simulink model "Gesamtmodell"  (R2017b)
settings: Solver=ode3  StartTime=0.0  StopTime=inf  FixedStep=dt  RelTol=1e-3  EnableMultiTasking=on
InitFcn:
  | Reglerauslegung
undefined symbols (not defined in the file or in its folder): aMax, aMaxPsi, Blindzeit, Com1, dt, K1, K2, K3, Kx, Ky, none, sigbuilder_block, Tx, Ty, vMax, vMaxPsi
libraries: xpcrtudplib x11, simulink x6, xpcutilitieslib x4, xpcseriallib x1, slrtlib x1
(part 1 of 4)
CloseFcn:
  | rtwprivate ssgencode ModelCloseRequest Robotino_Strecke_reall_2009
settings Model: SimulationMode=external  Creator=atlabor  LastModifiedBy=Robin
settings DataIOCC: SaveFormat=Array  SignalLoggingSaveFormat=ModelDataLogs
settings OptimizationCC: BlockReduction=off  OptimizeBlockIOStorage=off  BufferReuse=off  GlobalBufferReuse=off  ExpressionFolding=off  ExpressionDepthLimit=2147483647  LocalBlockOutputs=off  InitFltsAndDblsToZero=on  LifeSpan=inf
settings DebuggingCC: SaveWithParameterizedLinksMsg=none  UnderspecifiedInitializationDetection=Classic  MergeDetectMultiDrivingBlocksExec=none  SolverPrmCheckMsg=warning  FcnCallInpInsideContextMsg=warning  AllowSymbolicDim=off  StateNameClashWarn=warning  SFUnexpectedBacktrackingDiag=warning  SFNoUnconditionalDefaultTransitionDiag=warning  SFExecutionAtInitializationDiag=none
settings HardwareCC: ProdBitPerPointer=32  ProdBitPerSizeT=32  ProdBitPerPtrDiffT=32  ProdLargestAtomicFloat=None  ProdWordSize=32  ProdLongLongMode=on  ProdHWDeviceType=Generic->32-bit x86 compatible
settings ModelReferenceCC: PropagateSignalLabelsOutOfModel=off
settings SFSimCC: SimParseCustomCode=off
settings RTWCC: SystemTargetFile=slrt.tlc  TemplateMakefile=slrt_default_tmf  Description=Simulink Real-Time  CodeExecutionProfiling=on  RTWCompilerOptimization=on
settings CodeAppCC: StateflowObjectComments=on
settings ConfigComp: CovMetricSettings=dw  CovHtmlReporting=on  CovSaveCumulativeToWorkspaceVar=on  CovSaveSingleToWorkspaceVar=on  CovExternalEMLEnable=off  CovSFcnEnable=off

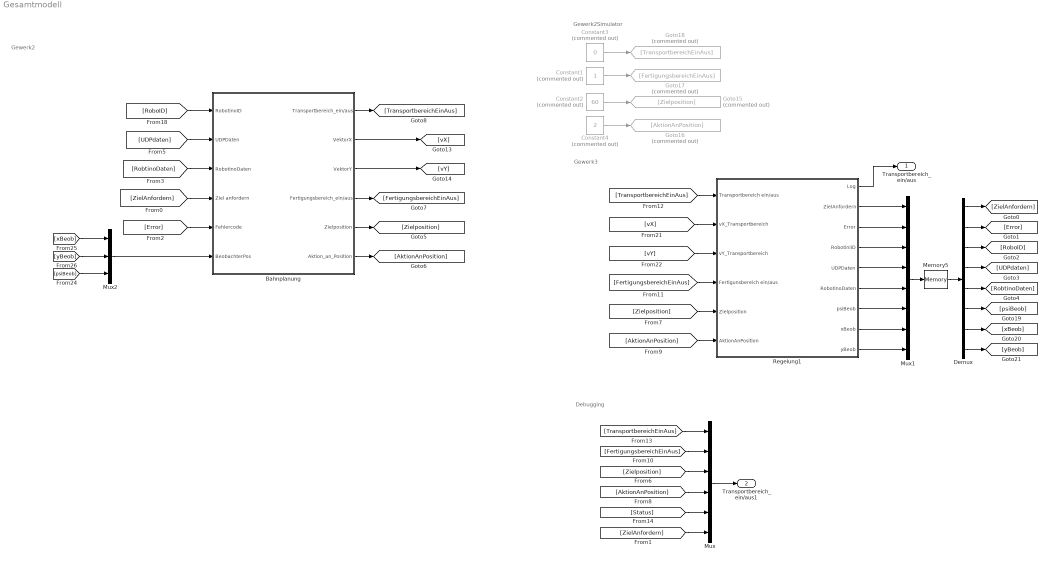
== system Gesamtmodell ==
  note: Gewerk2Simulator
  note: Gewerk3
  note: Gewerk2
  note: Debugging
  Bahnplanung : Subsystem
  Constant1 : Constant  Commented=on
  Constant2 : Constant  Commented=on  Value=60
  Constant3 : Constant  Commented=on  Value=0
  Constant4 : Constant  Commented=on  Value=2
  Demux : Demux  Outputs=8
  Goto15 : Goto  Commented=on  GotoTag=Zielposition
  Goto16 : Goto  Commented=on  GotoTag=AktionAnPosition
  Goto17 : Goto  Commented=on  GotoTag=FertigungsbereichEinAus
  Goto18 : Goto  Commented=on  GotoTag=TransportbereichEinAus
  Memory5 : Memory
  Mux : Mux  Inputs=6
  Mux1 : Mux  Inputs=8
  Mux2 : Mux  Inputs=3
  Regelung1 : Subsystem
  Transportbereich_ein/aus : Outport
  Transportbereich_ein/aus1 : Outport  Port=2
  wires:
  Regelung1/3(Error) -> Mux1/2
  Regelung1/6(RobotinoDaten) -> Mux1/5
  Regelung1/2(ZielAnfordern) -> Mux1/1
  Regelung1/4(RobotiniID) -> Mux1/3
  [ZielAnfordern] -> Mux/6
  Mux1/1 -> Memory5/1
  Demux/1 -> [ZielAnfordern]
  Demux/2 -> [Error]
  Memory5/1 -> Demux/1
  Demux/3 -> [RoboID]
  Demux/4 -> [UDPdaten]
  Regelung1/5(UDPDaten) -> Mux1/4
  Demux/5 -> [RobtinoDaten]
  [Zielposition] -> Mux/3
  [Zielposition] -> Regelung1/5(Zielposition)
  [AktionAnPosition] -> Mux/4
  [AktionAnPosition] -> Regelung1/6(AktionAnPosition)
  [FertigungsbereichEinAus] -> Mux/2
  [FertigungsbereichEinAus] -> Regelung1/4(Fertigunsbereich ein/aus)
  [TransportbereichEinAus] -> Regelung1/1(Transportbereich ein/aus)
  [TransportbereichEinAus] -> Mux/1
  [Status] -> Mux/5
  [vX] -> Regelung1/2(vX_Transportbereich)
  [vY] -> Regelung1/3(vY_Transportbereich)
  Constant3/1 -> Goto18/1
  Constant1/1 -> Goto17/1
  Constant2/1 -> Goto15/1
  Constant4/1 -> Goto16/1
  Regelung1/7(psiBeob) -> Mux1/6
  Regelung1/8(xBeob) -> Mux1/7
  Regelung1/9(yBeob) -> Mux1/8
  Demux/6 -> [psiBeob]
  Demux/7 -> [xBeob]
  Demux/8 -> [yBeob]
  [psiBeob] -> Mux2/3
  [xBeob] -> Mux2/1
  [yBeob] -> Mux2/2
  Regelung1/1(Log) -> Transportbereich_ein/aus/1
  Mux/1 -> Transportbereich_ein/aus1/1
  [UDPdaten] -> Bahnplanung/2(UDPDaten)
  [RobtinoDaten] -> Bahnplanung/3(RobotinoDaten)
  [ZielAnfordern] -> Bahnplanung/4(Ziel anfordern)
  [Error] -> Bahnplanung/5(Fehlercode)
  Mux2/1 -> Bahnplanung/6(BeobachterPos)
  Bahnplanung/1(Transportbereich_ein/aus) -> [TransportbereichEinAus]
  Bahnplanung/2(VektorX) -> [vX]
  Bahnplanung/3("VektorY ") -> [vY]
  Bahnplanung/4(Fertigungsbereich_ein/aus) -> [FertigungsbereichEinAus]
  Bahnplanung/5(Zielposition) -> [Zielposition]
  Bahnplanung/6(Aktion_an_Position) -> [AktionAnPosition]
  [RoboID] -> Bahnplanung/1(RobotinoID)

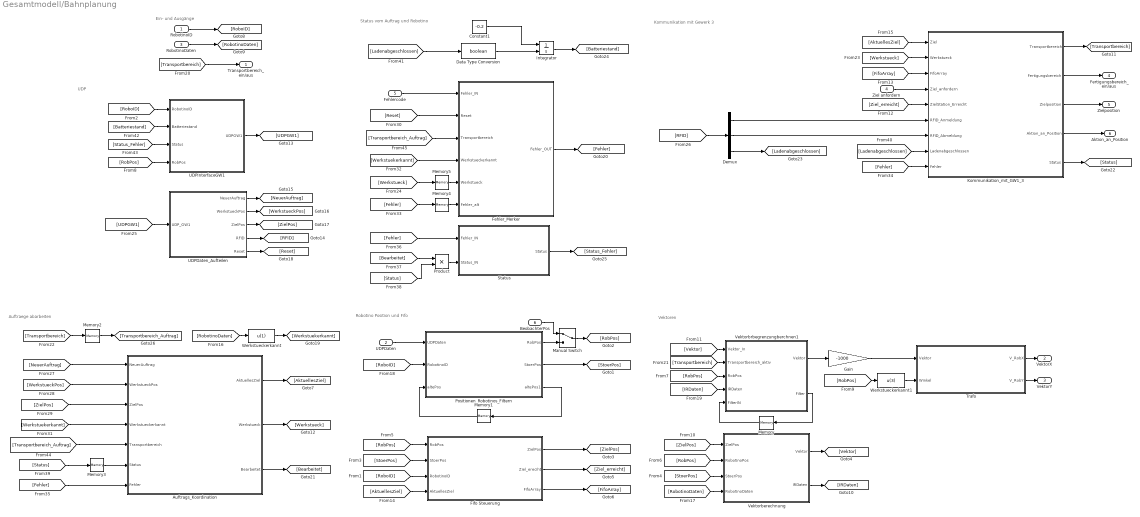
== system Gesamtmodell/Bahnplanung ==
  note: Ein- und Ausgänge
  note: Robotino Position und Fifo
  note: Status vom Auftrag und Robotino
  note: Auftraege abarbeiten
  note: Kommunikation mit Gewerk 3
  note: Vektoren
  note: UDP
  RobotinoID : Inport
  UDPDaten : Inport  Port=2  PortDimensions=56
  RobotinoDaten : Inport  Port=3
  Ziel anfordern : Inport  Port=4
  Fehlercode : Inport  Port=5
  BeobachterPos : Inport  Port=6
  Auftrags_Koordination : Stateflow chart  TreatAsAtomicUnit=on
  Constant1 : Constant  Value=-0.2
  Data Type Conversion : DataTypeConversion  OutDataTypeStr=boolean
  Demux : Demux  Outputs=3
  Fehler_Merker : MATLAB Function  TreatAsAtomicUnit=on
  Fifo Steuerung : Subsystem
  Gain : Gain  Gain=-1000
  Integrator : Integrator  ExternalReset=rising  InitialCondition=100  LimitOutput=on  UpperSaturationLimit=100  LowerSaturationLimit=0
  Kommunikation_mit_GW1_3 : Stateflow chart  TreatAsAtomicUnit=on
  Manual Switch : ManualSwitch
  Memory{,1..5} (6 alike) : Memory
  Positionen_Robotinos_Filtern : MATLAB Function  TreatAsAtomicUnit=on
  Product : Product
  Status : MATLAB Function  TreatAsAtomicUnit=on
  Trafo : MATLAB Function  Tag=Transformation_Global_auf_lokal  TreatAsAtomicUnit=on
  UDPDaten_Aufteilen : Subsystem
  UDPInterfaceGW1 : Subsystem
  Vektorberechnung : Subsystem
  Vektorbrbegrenzungberchnen1 : MATLAB Function  TreatAsAtomicUnit=on
  Werkstueckerkannt : Fcn  Expr=u(1)
  Werkstueckerkannt1 : Fcn  Expr=u(3)
  Transportbereich_ein/aus : Outport
  VektorX : Outport  Port=2  OutDataTypeStr=double
  "VektorY " : Outport  Port=3  OutDataTypeStr=double
  Fertigungsbereich_ein/aus : Outport  Port=4
  Zielposition : Outport  Port=5
  Aktion_an_Position : Outport  Port=6
  wires:
  Memory5/1 -> Fehler_Merker/5(Werkstueck)
  Memory4/1 -> Fehler_Merker/6(Fehler_alt)
  Data Type Conversion/1 -> Integrator/2
  Constant1/1 -> Integrator/1
  Fehlercode/1 -> Fehler_Merker/1(Fehler_IN)
  Memory1/1 -> Positionen_Robotinos_Filtern/3(altePos)
  Positionen_Robotinos_Filtern/3(altePos1) -> Memory1/1
  Memory/1 -> Vektorbrbegrenzungberchnen1/5(FilterIN)
  Demux/2 -> Kommunikation_mit_GW1_3/7(RFID_Abmeldung)
  Demux/1 -> Kommunikation_mit_GW1_3/6(RFID_Anmeldung)
  Ziel anfordern/1 -> Kommunikation_mit_GW1_3/4(Ziel_anfordern)
  Werkstueckerkannt1/1 -> Trafo/2(Winkel)
  BeobachterPos/1 -> Manual Switch/1
  Trafo/2(V_RobY) -> "VektorY "/1
  Trafo/1(V_RobX) -> VektorX/1
  Positionen_Robotinos_Filtern/1(RobPos) -> Manual Switch/2
  Gain/1 -> Trafo/1(Vektor)
  Vektorbrbegrenzungberchnen1/1(Vektor) -> Gain/1
  Kommunikation_mit_GW1_3/2(Fertigungsbereich) -> Fertigungsbereich_ein/aus/1
  Kommunikation_mit_GW1_3/4(Aktion_an_Position) -> Aktion_an_Position/1
  Kommunikation_mit_GW1_3/3(Zielposition) -> Zielposition/1
  UDPDaten/1 -> Positionen_Robotinos_Filtern/1(UDPDaten)
  [RoboID] -> Positionen_Robotinos_Filtern/2(RobotinoID)
  Memory3/1 -> Auftrags_Koordination/6(Status)
  RobotinoID/1 -> [RoboID]
  [RoboID] -> Fifo Steuerung/3(RobotinoID)
  [RoboID] -> UDPInterfaceGW1/1(RobotinoID)
  [StoerPos] -> Fifo Steuerung/2(StoerPos)
  [StoerPos] -> Vektorberechnung/3(StoerPos)
  Positionen_Robotinos_Filtern/2(StoerPos) -> [StoerPos]
  [RobPos] -> Fifo Steuerung/1(RobPos)
  [RobPos] -> Vektorberechnung/2(RobotinoPos)
  [RobPos] -> Vektorbrbegrenzungberchnen1/3(RobPos)
  [RobPos] -> UDPInterfaceGW1/4(RobPos)
  [RobPos] -> Werkstueckerkannt1/1
  Manual Switch/1 -> [RobPos]
  Fifo Steuerung/1(ZielPos) -> [ZielPos]
  [ZielPos] -> Vektorberechnung/1(ZielPos)
  Vektorberechnung/1(Vektor) -> [Vektor]
  [Vektor] -> Vektorbrbegrenzungberchnen1/1(Vektor_In)
  [Ziel_erreicht] -> Kommunikation_mit_GW1_3/5(ZielStation_Erreicht)
  Fifo Steuerung/2(Ziel_ereciht) -> [Ziel_erreicht]
  [FifoArray] -> Kommunikation_mit_GW1_3/3(FifoArray)
  Fifo Steuerung/3("FifoArray ") -> [FifoArray]
  [AktuellesZiel] -> Fifo Steuerung/4(AktuellesZiel)
  [AktuellesZiel] -> Kommunikation_mit_GW1_3/1(Ziel)
  Auftrags_Koordination/1(AktuellesZiel) -> [AktuellesZiel]
  [RobotinoDaten] -> Werkstueckerkannt/1
  [RobotinoDaten] -> Vektorberechnung/4(RobotinoDaten)
  RobotinoDaten/1 -> [RobotinoDaten]
  [IRDaten] -> Vektorbrbegrenzungberchnen1/4(IRDaten)
  Vektorberechnung/2(IRDaten) -> [IRDaten]
  [Transportbereich] -> Transportbereich_ein/aus/1
  [Transportbereich] -> Vektorbrbegrenzungberchnen1/2(Transportbereich_aktiv)
  [Transportbereich] -> Memory2/1
  Kommunikation_mit_GW1_3/1(Transportbereich) -> [Transportbereich]
  [Werkstueck] -> Kommunikation_mit_GW1_3/2(Werkstueck)
  [Werkstueck] -> Memory5/1
  Auftrags_Koordination/2(Werkstueck) -> [Werkstueck]
  [UDPGW1] -> UDPDaten_Aufteilen/1(UDP_GW1)
  UDPInterfaceGW1/1(UDPGW1) -> [UDPGW1]
  [RFID] -> Demux/1
  UDPDaten_Aufteilen/4(RFID) -> [RFID]
  [NeuerAuftrag] -> Auftrags_Koordination/1(NeuerAuftrag)
  UDPDaten_Aufteilen/1(NeuerAuftrag) -> [NeuerAuftrag]
  [WerkstueckPos] -> Auftrags_Koordination/2(WerkstueckPos)
  UDPDaten_Aufteilen/2(WerkstueckPos) -> [WerkstueckPos]
  [ZielPos] -> Auftrags_Koordination/3(ZielPos)
  UDPDaten_Aufteilen/3(ZielPos) -> [ZielPos]
  [Reset] -> Fehler_Merker/2(Reset)
  UDPDaten_Aufteilen/5(Reset) -> [Reset]
  [Werkstuekerkannt] -> Auftrags_Koordination/4(Werkstueckerkannt)
  [Werkstuekerkannt] -> Fehler_Merker/4(Werkstueckerkannt)
  Werkstueckerkannt/1 -> [Werkstuekerkannt]
  [Fehler] -> Memory4/1
  [Fehler] -> Kommunikation_mit_GW1_3/9(Fehler)
  [Fehler] -> Auftrags_Koordination/7(Fehler)
  [Fehler] -> Status/1(Fehler_IN)
  Fehler_Merker/1(Fehler_OUT) -> [Fehler]
  [Bearbeitet] -> Product/1
  [Status] -> Product/2
  [Status] -> Memory3/1
  Kommunikation_mit_GW1_3/5(Status) -> [Status]
  Auftrags_Koordination/3(Bearbeitet) -> [Bearbeitet]
  Product/1 -> Status/2(Status_IN)
  [Ladenabgeschlossen] -> Data Type Conversion/1
  [Ladenabgeschlossen] -> Kommunikation_mit_GW1_3/8(Ladenabgeschlossen)
  Demux/3 -> [Ladenabgeschlossen]
  [Batteriestand] -> UDPInterfaceGW1/2(Batteriestand)
  Integrator/1 -> [Batteriestand]
  [Status_Fehler] -> UDPInterfaceGW1/3(Status)
  Status/1(Status) -> [Status_Fehler]
  [Transportbereich_Auftrag] -> Fehler_Merker/3(Transportbereich)
  [Transportbereich_Auftrag] -> Auftrags_Koordination/5(Transportbereich)
  Memory2/1 -> [Transportbereich_Auftrag]
  Vektorbrbegrenzungberchnen1/2(Filter) -> Memory/1

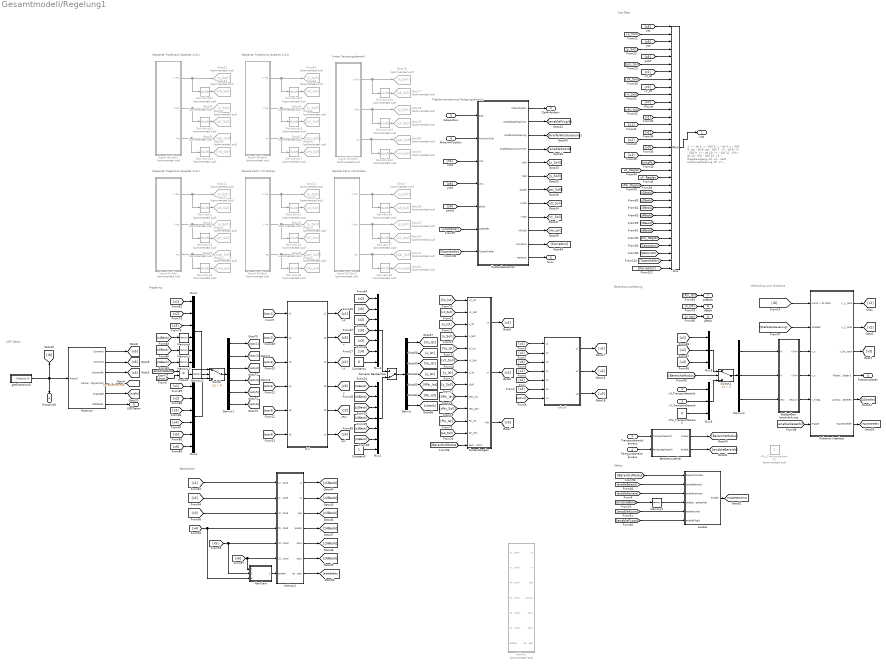
== system Gesamtmodell/Regelung1 ==
  note: Bereichsumschaltung
  note: Verbindung zum Robotino
  note: UDP Daten
  note: Geplante Trajektorie Quadrat 1x1m
  note: Log Data
  note: 1:    x     - Ist
      | 2:    x     - Soll
      | 3:    y     - Ist
      | 4:    y     - Soll
      | 5:   psi   - Ist
      | 6:   psi   - Soll
      | 7:   vX   - Ist
      | 8:   vX   - Soll
      | 9:   vY   - Ist
      | 10: vY   - Soll
      | 11: vPsi - Ist
      | 12: vPsi - Soll
      | 13: vX   - Reglerausgang
      | 14: vX   - nach InputLinearisierung
      | 15: vY   - Reglerausgang
      | 16: vY  - nach InputLinearisierung
      | 17: vPsi - Reglerausgang
      | 18: vPsi - nach InputLinearisierung
      | 19: Kamera Psi
      | 20: vX   - Regler (Geschwindigkeit)
      | 21: vY   - Regler (Geschwindigkeit)
      | 22: vPsi - Regler (Geschwindigkeit)
  note: Gerade Fahrt mit Drehen
  note: Gerade Fahrt mit Drehen
  note: Geplante Trajektorie Quadrat 1x1m
  note: Geplante Trajektorie Quadrat 1x1m
  note: hinter Fertigungsbereich
  note: Beobachter
  note: Regelung
  note: Trajektorienplanung Fertigungsbereich
  note: Safety
  Transportbereich ein/aus : Inport
  vX_Transportbereich : Inport  Port=2
  vY_Transportbereich : Inport  Port=3
  Fertigunsbereich ein/aus : Inport  Port=4
  Zielposition : Inport  Port=5
  AktionAnPosition : Inport  Port=6
  Bereichswaehler : MATLAB Function  TreatAsAtomicUnit=on
  Constant3 : Constant
  Constant4 : Constant  Value=0
  Demux : Demux  Outputs=7
  Demux1 : Demux  Outputs=6
  Demux2 : Demux  Outputs=3
  Derivative{,1..8,12..20} (18 alike) : Derivative  Commented=on
  Goto{11,21,27,52,63,76} (6 alike) : Goto  Commented=on  GotoTag=x_Soll
  Goto{12,22,28,53,64,77} (6 alike) : Goto  Commented=on  GotoTag=vX_Soll
  Goto{13,23,29,54,65,78} (6 alike) : Goto  Commented=on  GotoTag=y_Soll
  Goto{14,24,30,55,66,79} (6 alike) : Goto  Commented=on  GotoTag=vY_Soll
  Goto{15,25,31,56,67,80} (6 alike) : Goto  Commented=on  GotoTag=psi_Soll
  Goto{16,26,32,68..69,81} (6 alike) : Goto  Commented=on  GotoTag=vPsi_Soll
  Kalman : MATLAB Function  Commented=on  TreatAsAtomicUnit=on
  Kalman1 : MATLAB Function  TreatAsAtomicUnit=on
  Kamera/ Beobachter : ManualSwitch  CurrentSetting=0
  Memory{1..5} (5 alike) : Memory
  Mux : Mux  Inputs=33
  Mux1 : Mux  Inputs=7
  Mux2 : Mux  Inputs=6
  Mux3 : Mux  Inputs=7
  Mux4 : Mux  Inputs=6
  Mux5 : Mux  Inputs=3
  Mux6 : Mux  Inputs=3
  NewCam : MATLAB Function  TreatAsAtomicUnit=on
  Product : Product
  Receiver : Subsystem
  Robotino interface : Subsystem
  Signal Builder : Subsystem  Tag=STV Subsys  Commented=on  LoadFcn=sigbuilder_block('load');  StartFcn=sigbuilder_block('start');  StopFcn=sigbuilder_block('stop');  ClipboardFcn=sigbuilder_block('clipboard');  mask(Sigbuilder block){tuvar=[0:10]}
      mask help: Simulink:masks:SigbuilderBlock_MD
      mask init:
      | if ~strcmp(get_param(bdroot(gcbh),'SimulationStatus'),'stopped') tuvar = sigbuilder_block('maskInit'); end
      settings: CopyFcn=sigbuilder_block('copy');  DeleteFcn=sigbuilder_block('delete');  ModelCloseFcn=sigbuilder_block('modelClose');  PreSaveFcn=sigbuilder_block('preSave');  PauseFcn=sigbuilder_block('pause');  ContinueFcn=sigbuilder_block('continue');  NameChangeFcn=sigbuilder_block('namechange');  OpenFcn=sigbuilder_block('open',[6 30 1248 660 ]);  CloseFcn=sigbuilder_block('close');
      mask Display: plot(0, 0, 100, 100,[2, 2, 32, 32, 2], [68, 8, 8, 68, 68],[32, 2], [38, 38], [32, 19, 2],[53, 60, 44], [32, 17, 17, 2],[16, 16, 31, 31]);txt = getActiveGroup(gcbh);text(2, 100, txt,'verticalAlignment', 'top');
  Signal Builder1 : Subsystem  Tag=STV Subsys  Commented=on  LoadFcn=sigbuilder_block('load');  StartFcn=sigbuilder_block('start');  StopFcn=sigbuilder_block('stop');  ClipboardFcn=sigbuilder_block('clipboard');  mask(Sigbuilder block){tuvar=[0:10]}
      mask help: Simulink:masks:SigbuilderBlock_MD
      mask init:
      | if ~strcmp(get_param(bdroot(gcbh),'SimulationStatus'),'stopped') tuvar = sigbuilder_block('maskInit'); end
      settings: CopyFcn=sigbuilder_block('copy');  DeleteFcn=sigbuilder_block('delete');  ModelCloseFcn=sigbuilder_block('modelClose');  PreSaveFcn=sigbuilder_block('preSave');  PauseFcn=sigbuilder_block('pause');  ContinueFcn=sigbuilder_block('continue');  NameChangeFcn=sigbuilder_block('namechange');  OpenFcn=sigbuilder_block('open',[6.06316 30.3158 1248.25 659.368 ]);  CloseFcn=sigbuilder_block('close');
      mask Display: plot(0, 0, 100, 100,[2, 2, 32, 32, 2], [68, 8, 8, 68, 68],[32, 2], [38, 38], [32, 19, 2],[53, 60, 44], [32, 17, 17, 2],[16, 16, 31, 31]);txt = getActiveGroup(gcbh);text(2, 100, txt,'verticalAlignment', 'top');
  Signal Builder2 : Subsystem  Tag=STV Subsys  Commented=on  LoadFcn=sigbuilder_block('load');  StartFcn=sigbuilder_block('start');  StopFcn=sigbuilder_block('stop');  ClipboardFcn=sigbuilder_block('clipboard');  mask(Sigbuilder block){tuvar=[0:10]}
      mask help: Simulink:masks:SigbuilderBlock_MD
      mask init:
      | if ~strcmp(get_param(bdroot(gcbh),'SimulationStatus'),'stopped') tuvar = sigbuilder_block('maskInit'); end
      settings: CopyFcn=sigbuilder_block('copy');  DeleteFcn=sigbuilder_block('delete');  ModelCloseFcn=sigbuilder_block('modelClose');  PreSaveFcn=sigbuilder_block('preSave');  PauseFcn=sigbuilder_block('pause');  ContinueFcn=sigbuilder_block('continue');  NameChangeFcn=sigbuilder_block('namechange');  OpenFcn=sigbuilder_block('open',[6 30 1248 660 ]);  CloseFcn=sigbuilder_block('close');
      mask Display: plot(0, 0, 100, 100,[2, 2, 32, 32, 2], [68, 8, 8, 68, 68],[32, 2], [38, 38], [32, 19, 2],[53, 60, 44], [32, 17, 17, 2],[16, 16, 31, 31]);txt = getActiveGroup(gcbh);text(2, 100, txt,'verticalAlignment', 'top');
  Signal Builder3 : Subsystem  Tag=STV Subsys  Commented=on  LoadFcn=sigbuilder_block('load');  StartFcn=sigbuilder_block('start');  StopFcn=sigbuilder_block('stop');  ClipboardFcn=sigbuilder_block('clipboard');  mask(Sigbuilder block){tuvar=[0:10]}
      mask help: Simulink:masks:SigbuilderBlock_MD
      mask init:
      | if ~strcmp(get_param(bdroot(gcbh),'SimulationStatus'),'stopped') tuvar = sigbuilder_block('maskInit'); end
      settings: CopyFcn=sigbuilder_block('copy');  DeleteFcn=sigbuilder_block('delete');  ModelCloseFcn=sigbuilder_block('modelClose');  PreSaveFcn=sigbuilder_block('preSave');  PauseFcn=sigbuilder_block('pause');  ContinueFcn=sigbuilder_block('continue');  NameChangeFcn=sigbuilder_block('namechange');  OpenFcn=sigbuilder_block('open',[6 30 1248 660 ]);  CloseFcn=sigbuilder_block('close');
      mask Display: plot(0, 0, 100, 100,[2, 2, 32, 32, 2], [68, 8, 8, 68, 68],[32, 2], [38, 38], [32, 19, 2],[53, 60, 44], [32, 17, 17, 2],[16, 16, 31, 31]);txt = getActiveGroup(gcbh);text(2, 100, txt,'verticalAlignment', 'top');
  Signal Builder4 : Subsystem  Tag=STV Subsys  Commented=on  LoadFcn=sigbuilder_block('load');  StartFcn=sigbuilder_block('start');  StopFcn=sigbuilder_block('stop');  ClipboardFcn=sigbuilder_block('clipboard');  mask(Sigbuilder block){tuvar=[0:10]}
      mask help: Simulink:masks:SigbuilderBlock_MD
      mask init:
      | if ~strcmp(get_param(bdroot(gcbh),'SimulationStatus'),'stopped') tuvar = sigbuilder_block('maskInit'); end
      settings: CopyFcn=sigbuilder_block('copy');  DeleteFcn=sigbuilder_block('delete');  ModelCloseFcn=sigbuilder_block('modelClose');  PreSaveFcn=sigbuilder_block('preSave');  PauseFcn=sigbuilder_block('pause');  ContinueFcn=sigbuilder_block('continue');  NameChangeFcn=sigbuilder_block('namechange');  OpenFcn=sigbuilder_block('open',[6 30 1248 660 ]);  CloseFcn=sigbuilder_block('close');
      mask Display: plot(0, 0, 100, 100,[2, 2, 32, 32, 2], [68, 8, 8, 68, 68],[32, 2], [38, 38], [32, 19, 2],[53, 60, 44], [32, 17, 17, 2],[16, 16, 31, 31]);txt = getActiveGroup(gcbh);text(2, 100, txt,'verticalAlignment', 'top');
  Signal Builder5 : Subsystem  Tag=STV Subsys  Commented=on  LoadFcn=sigbuilder_block('load');  StartFcn=sigbuilder_block('start');  StopFcn=sigbuilder_block('stop');  ClipboardFcn=sigbuilder_block('clipboard');  mask(Sigbuilder block){tuvar=[0:10]}
      mask help: Simulink:masks:SigbuilderBlock_MD
      mask init:
      | if ~strcmp(get_param(bdroot(gcbh),'SimulationStatus'),'stopped') tuvar = sigbuilder_block('maskInit'); end
      settings: CopyFcn=sigbuilder_block('copy');  DeleteFcn=sigbuilder_block('delete');  ModelCloseFcn=sigbuilder_block('modelClose');  PreSaveFcn=sigbuilder_block('preSave');  PauseFcn=sigbuilder_block('pause');  ContinueFcn=sigbuilder_block('continue');  NameChangeFcn=sigbuilder_block('namechange');  OpenFcn=sigbuilder_block('open',[6 30 1248 660 ]);  CloseFcn=sigbuilder_block('close');
      mask Display: plot(0, 0, 100, 100,[2, 2, 32, 32, 2], [68, 8, 8, 68, 68],[32, 2], [38, 38], [32, 19, 2],[53, 60, 44], [32, 17, 17, 2],[16, 16, 31, 31]);txt = getActiveGroup(gcbh);text(2, 100, txt,'verticalAlignment', 'top');
  "Stellgrößen- beschränkung " : Subsystem
  Switch : Switch  Criteria=u2 > Threshold
  Switch1 : Switch  Criteria=u2 > Threshold
  Zustandsautomat : Subsystem
  Zustandsregler : Subsystem
  "enable " : MATLAB Function  TreatAsAtomicUnit=on
  getRobotinoID : Subsystem
  "u(x,v) " : MATLAB Function  TreatAsAtomicUnit=on
  vPsi_Transportbereich : Constant  Value=0
  vPsi_Transportbereich1 : Constant  Commented=on
  z(x) : MATLAB Function  TreatAsAtomicUnit=on
  Log : Outport
  ZielAnfordern : Outport  Port=2
  Error : Outport  Port=3
  RobotiniID : Outport  Port=4
  UDPDaten : Outport  Port=5
  RobotinoDaten : Outport  Port=6
  psiBeob : Outport  Port=7
  xBeob : Outport  Port=8
  yBeob : Outport  Port=9
  wires:
  [Korrektur] -> Mux/33
  Zustandsautomat/11(Korrektur) -> [Korrektur]
  [enableGewerk3] -> Robotino interface/6(enable)
  "enable "/1(enable) -> [enableGewerk3]
  [enableFLogik] -> "enable "/6(enableFlogik)
  [enableKoord] -> "enable "/5(enableKoord)
  [BereichsModus] -> "enable "/1(BereichsModus)
  [enableBereich] -> "enable "/2(enableBereich)
  [enableKamera] -> "enable "/3(enableKamera)
  Memory5/1 -> "enable "/4(enableBeobachter)
  [enableBeob] -> Memory5/1
  [LSGreifer] -> Zustandsautomat/6("LSGreifer ")
  Robotino interface/5(LichtschrankeGreifer) -> [LSGreifer]
  [BereichsModus] -> Zustandsregler/13(Fertigungsbereich Aktiv)
  [BereichsModus] -> Switch1/2
  Bereichswaehler/1(modus) -> [BereichsModus]
  [StationsNr] -> Mux/31
  [Zielposition] -> Mux/30
  Fertigunsbereich ein/aus/1 -> Bereichswaehler/2(fertigungsbereich)
  Bereichswaehler/2(enable) -> [enableBereich]
  Zustandsautomat/12(FehlerNr) -> Error/1
  Mux5/1 -> Switch1/1
  [u1] -> Mux5/1
  [GreiferAnsteuerung] -> Robotino interface/2(Grabber)
  Mux/1 -> Log/1
  Derivative4/1 -> Goto16/1
  Signal Builder/1(X Pos) -> Derivative/1, Goto11/1
  [u2] -> Mux5/2
  [u3] -> Mux5/3
  vPsi_Transportbereich/1 -> Mux6/3
  Transportbereich ein/aus/1 -> Bereichswaehler/1(transportbereich)
  Mux6/1 -> Switch1/3
  [z1] -> Mux/7
  [u2] -> Mux/16
  Receiver/5("origAngle ") -> [origPsi]
  Demux2/2 -> "Stellgrößen- beschränkung "/2(vY)
  Demux2/3 -> "Stellgrößen- beschränkung "/3(vPsi)
  Signal Builder5/3(Psi) -> Goto80/1, Derivative20/1
  [u3] -> Mux/18
  [u1] -> Mux/14
  Signal Builder1/1(X Pos) -> Derivative1/1, Goto21/1
  [origPsi] -> Mux/19
  [z5] -> Mux/1
  "Stellgrößen- beschränkung "/1(vXlim) -> Robotino interface/3(v_x)
  Signal Builder2/3(Psi) -> Derivative8/1, Goto31/1
  Derivative7/1 -> Goto30/1
  Signal Builder3/3(Psi) -> Goto56/1, Derivative14/1
  Signal Builder1/2(Y Pos) -> Derivative2/1, Goto23/1
  [v3] -> Mux/17
  Receiver/4(CameraSignalValid) -> [enableKamera]
  [z6] -> Mux/3
  Receiver/3("CameraPsi ") -> [x4]
  [vPsi_Soll] -> Mux/12
  vX_Transportbereich/1 -> Mux6/1
  [z2Beob] -> Mux/24
  [z6Beob] -> Mux/28
  [vY_Soll] -> Mux/10
  [vX_Soll] -> Mux/8
  Signal Builder4/3(Psi) -> Goto67/1, Derivative17/1
  Robotino interface/3("v_Psi_lokal ") -> [x3]
  Robotino interface/2("v_Y_lokal ") -> [x2]
  [z3] -> Mux/11
  [z2] -> Mux/9
  [z3Beob] -> Mux/25
  vY_Transportbereich/1 -> Mux6/2
  [ID] -> Robotino interface/1(number of robot)
  Signal Builder3/2(Y Pos) -> Goto54/1, Derivative13/1
  Derivative/1 -> Goto12/1
  [vY_Regler] -> Mux/21
  "Stellgrößen- beschränkung "/3(vPsiLim) -> Robotino interface/5(v_theta)
  AktionAnPosition/1 -> Zustandsautomat/2(AktionAnZiel)
  [z4Beob] -> Mux/26
  [z5Beob] -> Mux/27
  Signal Builder4/1(X Pos) -> Goto63/1, Derivative15/1
  Zielposition/1 -> Zustandsautomat/1("Ziel ")
  Signal Builder4/2(Y Pos) -> Goto65/1, Derivative16/1
  Receiver/1(CameraX) -> [x5]
  Receiver/2(CameraY) -> [x6]
  [x_Soll] -> Mux/2
  Signal Builder3/1(X Pos) -> Goto52/1, Derivative12/1
  Robotino interface/1(v_X_lokal) -> [x1]
  "Stellgrößen- beschränkung "/2(vYlim) -> Robotino interface/4(v_y)
  Derivative18/1 -> Goto77/1
  Derivative19/1 -> Goto79/1
  Derivative20/1 -> Goto81/1
  Derivative12/1 -> Goto53/1
  Derivative14/1 -> Goto69/1
  Derivative8/1 -> Goto32/1
  [vPsi_Regler] -> Mux/22
  Signal Builder/2(Y Pos) -> Derivative3/1, Goto13/1
  Signal Builder5/1(X Pos) -> Goto76/1, Derivative18/1
  [psi_Soll] -> Mux/6
  [v1] -> Mux/13
  [v2] -> Mux/15
  Derivative15/1 -> Goto64/1
  Derivative17/1 -> Goto68/1
  Derivative16/1 -> Goto66/1
  Derivative13/1 -> Goto55/1
  [z1Beob] -> Mux/23
  Derivative2/1 -> Goto24/1
  Signal Builder/3(Psi) -> Derivative4/1, Goto15/1
  Derivative3/1 -> Goto14/1
  getRobotinoID/1(Robotino.ID) -> RobotiniID/1, [ID], Receiver/1("RoboID ")
  Derivative6/1 -> Goto28/1
  Signal Builder2/2(Y Pos) -> Derivative7/1, Goto29/1
  Signal Builder5/2(Y Pos) -> Goto78/1, Derivative19/1
  Derivative5/1 -> Goto26/1
  Demux2/1 -> "Stellgrößen- beschränkung "/1(vX)
  Signal Builder2/1(X Pos) -> Derivative6/1, Goto27/1
  Signal Builder1/3(Psi) -> Derivative5/1, Goto25/1
  Derivative1/1 -> Goto22/1
  [y_Soll] -> Mux/4
  [z4] -> Mux/5
  [vX_Regler] -> Mux/20
  Receiver/6(UDPDaten) -> UDPDaten/1
  Robotino interface/4(RobotinoDaten 1) -> RobotinoDaten/1
  Switch1/1 -> Demux2/1
  Kalman1/2(vy) -> [z2Beob]
  [z3] -> Kalman1/3(vPsiZustand)
  Constant4/1 -> Mux3/7
  [x4] -> Mux4/4
  Demux1/1 -> [actx1]
  Demux/1 -> [Vx_Ist]
  [z2] -> Kalman1/2(vyZustand)
  [x5] -> NewCam/2(xZustand), Kalman1/5(xZustand)
  Zustandsregler/2(vY) -> [v2]
  [x4] -> NewCam/3(psiZustand), Kalman1/4(PsiZustand)
  [z1Beob] -> Mux1/1
  [z5Beob] -> Memory3/1
  [z2Beob] -> Mux1/3
  [x1] -> "u(x,v) "/4(x1)
  [actx3] -> z(x)/3(x3)
  "u(x,v) "/3(u3) -> [u3]
  [z5] -> Mux3/2
  Kalman1/5(posx) -> [z5Beob]
  Memory3/1 -> Mux2/5
  [z3Beob] -> Mux1/5
  [vX_Soll] -> Zustandsregler/2("vX_Soll ")
  [x2] -> Mux4/2
  [z1] -> Kalman1/1(vxZustand)
  [check] -> Product/2
  NewCam/1(enable) -> Kalman1/7(enable)
  Demux/3 -> [Vy_Ist]
  [x1] -> Mux4/1
  Memory2/1 -> Mux2/6
  [enableBeob] -> Product/1
  [z2] -> Mux3/3
  Kalman1/6(posy) -> [z6Beob]
  [v1] -> "u(x,v) "/1(v1)
  [z4] -> Mux3/6
  [actx4] -> "u(x,v) "/7(x4)
  [z6] -> Mux3/4
  [z1] -> Mux3/1
  Mux1/1 -> Kamera/ Beobachter/2
  [x3] -> Mux4/3
  [z6Beob] -> Mux1/4
  Kalman1/3(vpsi) -> [z3Beob]
  [x3] -> "u(x,v) "/6(x3)
  [VPsi_Ist] -> Zustandsregler/9(vPsi_ist)
  Demux/6 -> [Psi_Ist]
  "u(x,v) "/2(u2) -> [u2]
  Mux4/1 -> Switch/3
  [Psi_Ist] -> Zustandsregler/11(Psi_ist)
  [actx1] -> z(x)/1(x1)
  [x2] -> "u(x,v) "/5(x2)
  [z5Beob] -> Mux1/2
  [y_Ist] -> Zustandsregler/7(y_Ist)
  [x2] -> Mux2/2
  [v2] -> "u(x,v) "/2(v2)
  [v3] -> "u(x,v) "/3(v3)
  [Vy_Ist] -> Zustandsregler/5(vY_Ist)
  Zustandsregler/3("vPsi ") -> [v3]
  z(x)/1(z1) -> [z1]
  [x6] -> Mux4/6
  Kalman1/1(vx) -> [z1Beob]
  [z4Beob] -> Mux1/6
  z(x)/6(z4) -> [z4]
  Demux/7 -> [check]
  "u(x,v) "/1(u1) -> [u1]
  [x3] -> Mux2/3
  [actx2] -> z(x)/2(x2)
  [actx4] -> z(x)/4(x4)
  [x_Ist] -> Zustandsregler/3(x_Ist)
  Demux1/6 -> [actx6]
  [z3] -> Mux3/5
  Zustandsregler/1(vX) -> [v1]
  [vPsi_Soll] -> Zustandsregler/10(vPsi_Soll)
  [Vx_Ist] -> Zustandsregler/1(vX_Ist)
  Demux/2 -> [x_Ist]
  [psi_Soll] -> Zustandsregler/12("psi_Soll ")
  [z6Beob] -> Memory2/1
  Product/1 -> Memory1/1
  [vY_Soll] -> Zustandsregler/6("vY_Soll ")
  Demux1/5 -> [actx5]
  Demux1/4 -> [actx4]
  z(x)/3(z2) -> [z2]
  Demux/4 -> [y_Ist]
  [actx5] -> z(x)/5(x5)
  Kalman1/4(pospsi) -> [z4Beob]
  [z4Beob] -> Memory4/1
  Constant3/1 -> Mux1/7
  Kamera/ Beobachter/1 -> Demux/1
  [x1] -> Mux2/1
  [x5] -> Mux4/5
  Demux/5 -> [VPsi_Ist]
  z(x)/2(z5) -> [z5]
  Demux1/2 -> [actx2]
  z(x)/4(z6) -> [z6]
  Memory1/1 -> Switch/2
  Demux1/3 -> [actx3]
  Memory4/1 -> Mux2/4
  Mux2/1 -> Switch/1
  [y_Soll] -> Zustandsregler/8(ySoll)
  [x6] -> NewCam/1(yZustand), Kalman1/6(yZustand)
  [actx6] -> z(x)/6(x6)
  Kalman1/7(enableBeob) -> [enableBeob]
  z(x)/5(z3) -> [z3]
  Mux3/1 -> Kamera/ Beobachter/1
  Switch/1 -> Demux1/1
  [x_Soll] -> Zustandsregler/4(x_Soll)
  Zustandsautomat/3(GreiferAnsteuerung) -> [GreiferAnsteuerung]
  Zustandsautomat/7(psiSoll) -> [psi_Soll]
  Zustandsautomat/2(enableStateMachine) -> [enableFLogik]
  [z6] -> Zustandsautomat/4(yIst)
  Zustandsautomat/4(enableStationsnummer) -> [enableKoord]
  Zustandsautomat/10(vPsiSoll) -> [vPsi_Soll]
  Zustandsautomat/8(vXSoll) -> [vX_Soll]
  Zustandsautomat/5(xSoll) -> [x_Soll]
  Zustandsautomat/9(vYSoll) -> [vY_Soll]
  Zustandsautomat/6(YSoll) -> [y_Soll]
  [z5] -> Zustandsautomat/3(xIst)
  [z4] -> Zustandsautomat/5(psiIst)
  Zustandsautomat/1(ZielAnfordern) -> ZielAnfordern/1
  [Psi_Ist] -> psiBeob/1
  [x_Ist] -> xBeob/1
  [y_Ist] -> yBeob/1
  [pXI_Regler] -> Mux/29
  Robotino interface/6(TasterGreifer) -> [TasterGreifer]
  [TasterGreifer] -> Zustandsautomat/7("TasterGreifer ")
  [TasterGreifer] -> Mux/32

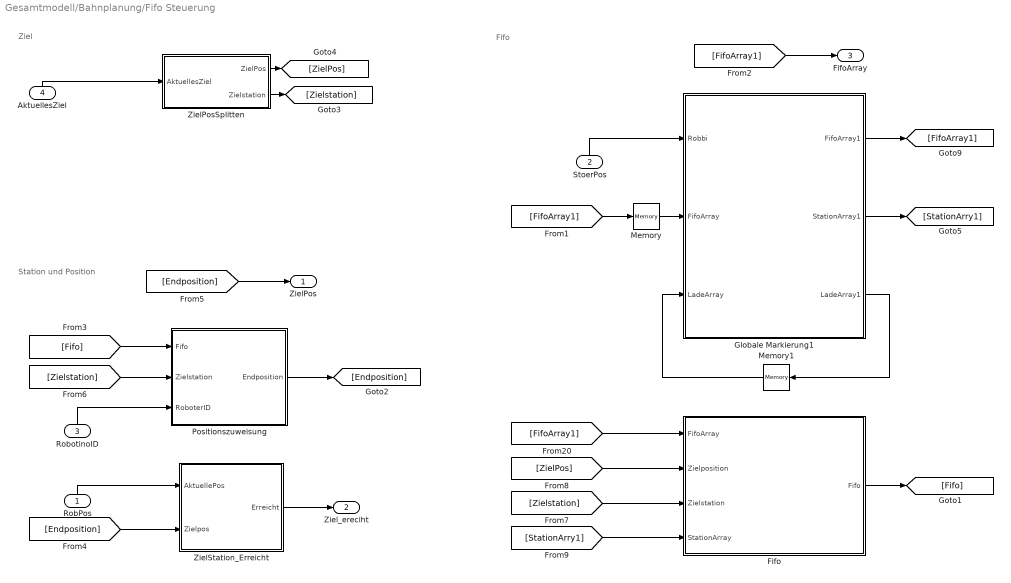
== system Gesamtmodell/Bahnplanung/Fifo Steuerung ==
  note: Ziel
  note: Fifo
  note: Station und Position
  RobPos : Inport  PortDimensions=3
  StoerPos : Inport  Port=2  PortDimensions=15
  RobotinoID : Inport  Port=3
  AktuellesZiel : Inport  Port=4
  Fifo : Stateflow chart  TreatAsAtomicUnit=on
  Globale Markierung1 : MATLAB Function  TreatAsAtomicUnit=on
  Memory : Memory
  Memory1 : Memory
  Positionszuweisung : MATLAB Function  TreatAsAtomicUnit=on
  ZielPosSplitten : MATLAB Function  TreatAsAtomicUnit=on
  ZielStation_Erreicht : MATLAB Function  TreatAsAtomicUnit=on
  ZielPos : Outport  PortDimensions=[1 2]
  Ziel_ereciht : Outport  Port=2
  "FifoArray " : Outport  Port=3
  wires:
  ZielStation_Erreicht/1(Erreicht) -> Ziel_ereciht/1
  Memory1/1 -> Globale Markierung1/3(LadeArray)
  Globale Markierung1/3(LadeArray1) -> Memory1/1
  Memory/1 -> Globale Markierung1/2(FifoArray)
  AktuellesZiel/1 -> ZielPosSplitten/1(AktuellesZiel)
  StoerPos/1 -> Globale Markierung1/1(Robbi)
  RobPos/1 -> ZielStation_Erreicht/1(AktuellePos)
  RobotinoID/1 -> Positionszuweisung/3(RoboterID)
  [FifoArray1] -> Fifo/1(FifoArray)
  [FifoArray1] -> Memory/1
  Globale Markierung1/1(FifoArray1) -> [FifoArray1]
  [FifoArray1] -> "FifoArray "/1
  [Fifo] -> Positionszuweisung/1(Fifo)
  Fifo/1(Fifo) -> [Fifo]
  [Endposition] -> ZielStation_Erreicht/2(Zielpos)
  [Endposition] -> ZielPos/1
  Positionszuweisung/1(Endposition) -> [Endposition]
  [Zielstation] -> Positionszuweisung/2(Zielstation)
  ZielPosSplitten/2(Zielstation) -> [Zielstation]
  [Zielstation] -> Fifo/3(Zielstation)
  [ZielPos] -> Fifo/2(Zielposition)
  ZielPosSplitten/1(ZielPos) -> [ZielPos]
  Globale Markierung1/2(StationArray1) -> [StationArry1]
  [StationArry1] -> Fifo/4(StationArray)

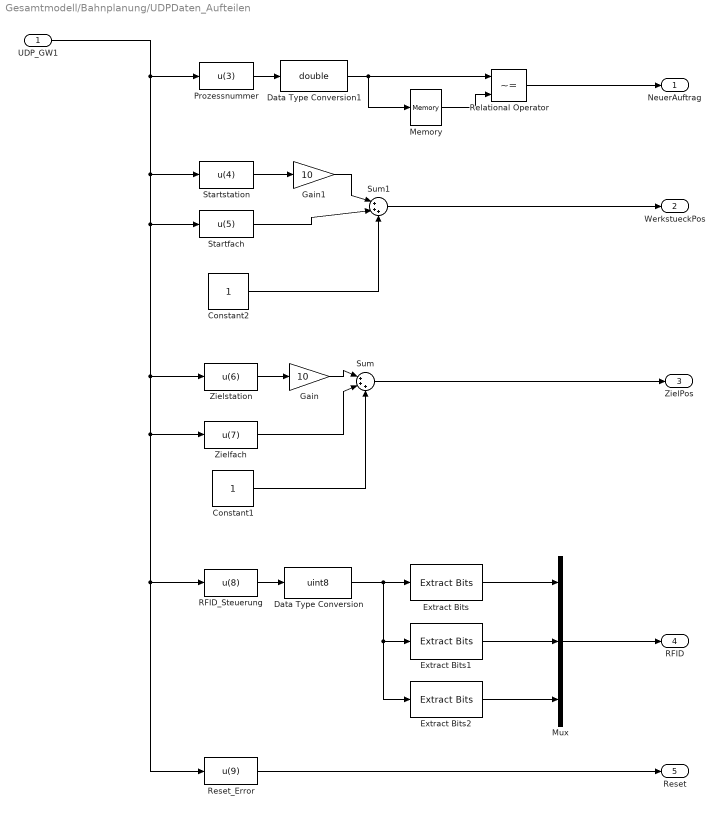
== system Gesamtmodell/Bahnplanung/UDPDaten_Aufteilen ==
  UDP_GW1 : Inport
  Constant1 : Constant
  Constant2 : Constant
  Data Type Conversion : DataTypeConversion  OutDataTypeStr=uint8
  Data Type Conversion1 : DataTypeConversion  OutDataTypeStr=double
  Extract Bits : simulink/Logic and Bit Operations/Extract Bits  bitsToExtract=Range of bits  numBits=8  bitIdxRange=[0]  outScalingMode=Treat bit field as an integer
      settings: SourceProductName=Simulink
  Extract Bits1 : simulink/Logic and Bit Operations/Extract Bits  bitsToExtract=Range of bits  numBits=8  bitIdxRange=[1]  outScalingMode=Treat bit field as an integer
      settings: SourceProductName=Simulink
  Extract Bits2 : simulink/Logic and Bit Operations/Extract Bits  bitsToExtract=Range of bits  numBits=8  bitIdxRange=[2]  outScalingMode=Treat bit field as an integer
      settings: SourceProductName=Simulink
  Gain : Gain  Gain=10
  Gain1 : Gain  Gain=10
  Memory : Memory
  Mux : Mux  Inputs=3
  Prozessnummer : Fcn  Expr=u(3)
  RFID_Steuerung : Fcn  Expr=u(8)
  Relational Operator : RelationalOperator  Operator=~=  OutDataTypeStr=boolean  RndMeth=Nearest
  Reset_Error : Fcn  Expr=u(9)
  Startfach : Fcn  Expr=u(5)
  Startstation : Fcn  Expr=u(4)
  Sum : Sum  Inputs=|+++
  Sum1 : Sum  Inputs=|+++
  Zielfach : Fcn  Expr=u(7)
  Zielstation : Fcn  Expr=u(6)
  NeuerAuftrag : Outport
  WerkstueckPos : Outport  Port=2
  ZielPos : Outport  Port=3
  RFID : Outport  Port=4
  Reset : Outport  Port=5
  wires:
  Reset_Error/1 -> Reset/1
  Extract Bits2/1 -> Mux/3
  Extract Bits/1 -> Mux/1
  Prozessnummer/1 -> Data Type Conversion1/1
  Mux/1 -> RFID/1
  Extract Bits1/1 -> Mux/2
  Memory/1 -> Relational Operator/2
  Data Type Conversion1/1 -> Relational Operator/1, Memory/1
  Data Type Conversion/1 -> Extract Bits/1, Extract Bits2/1, Extract Bits1/1
  RFID_Steuerung/1 -> Data Type Conversion/1
  Relational Operator/1 -> NeuerAuftrag/1
  Sum/1 -> ZielPos/1
  Constant1/1 -> Sum/3
  Startstation/1 -> Gain1/1
  Constant2/1 -> Sum1/3
  Gain1/1 -> Sum1/1
  Startfach/1 -> Sum1/2
  Sum1/1 -> WerkstueckPos/1
  UDP_GW1/1 -> RFID_Steuerung/1, Reset_Error/1, Zielfach/1, Zielstation/1, Startfach/1, Startstation/1, Prozessnummer/1
  Zielstation/1 -> Gain/1
  Gain/1 -> Sum/1
  Zielfach/1 -> Sum/2

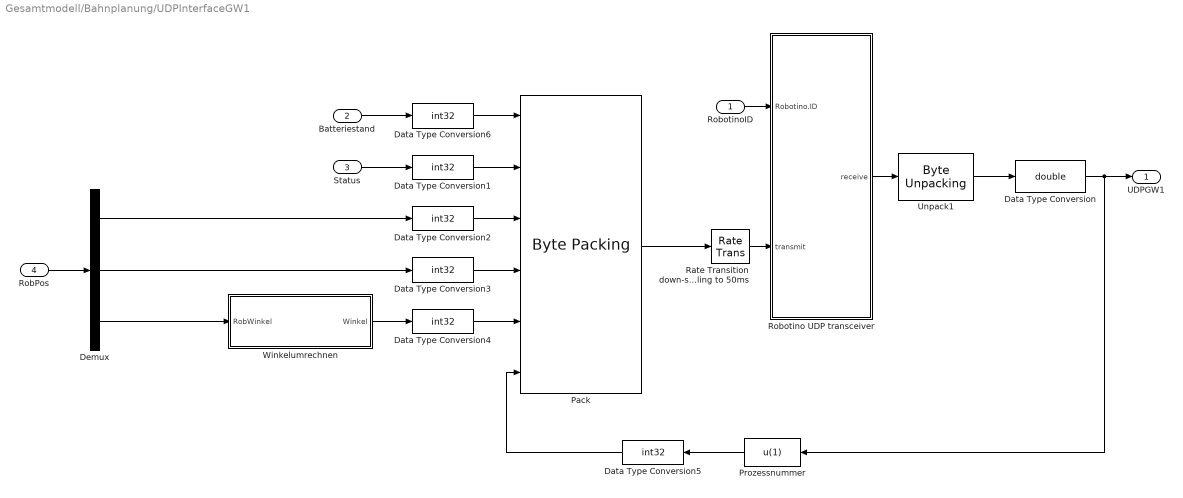
== system Gesamtmodell/Bahnplanung/UDPInterfaceGW1 ==
  RobotinoID : Inport
  Batteriestand : Inport  Port=2
  Status : Inport  Port=3
  RobPos : Inport  Port=4
  Data Type Conversion : DataTypeConversion  OutDataTypeStr=double
  Data Type Conversion{1..6} (6 alike) : DataTypeConversion  OutDataTypeStr=int32
  Demux : Demux  Outputs=3
  Pack : xpcutilitieslib/Byte Packing   MaskPackedDataType=uint8  MaskUnpackedDataTypes={'int32','int32','int32','int32','int32','int32'}  MaskAlignment=1
  Prozessnummer : Fcn  Expr=u(1)
  Rate Transition down-sampling to 50ms : RateTransition  OutPortSampleTime=0.05
  Robotino UDP transceiver : Subsystem
  Unpack1 : xpcutilitieslib/Byte Unpacking   MaskUnpackedDataTypes={'int32'}  MaskUnpackedDataSizes={[9]}  MaskAlignment=1
      settings: SourceProductName=Simulink Real-Time  SourceProductBaseCode=XP
  Winkelumrechnen : MATLAB Function  TreatAsAtomicUnit=on
  UDPGW1 : Outport
  wires:
  Data Type Conversion5/1 -> Pack/6
  Prozessnummer/1 -> Data Type Conversion5/1
  Winkelumrechnen/1(Winkel) -> Data Type Conversion4/1
  Demux/3 -> Winkelumrechnen/1(RobWinkel)
  Demux/2 -> Data Type Conversion3/1
  Demux/1 -> Data Type Conversion2/1
  RobPos/1 -> Demux/1
  Data Type Conversion4/1 -> Pack/5
  Data Type Conversion3/1 -> Pack/4
  Data Type Conversion2/1 -> Pack/3
  Data Type Conversion/1 -> UDPGW1/1, Prozessnummer/1
  Unpack1/1 -> Data Type Conversion/1
  RobotinoID/1 -> Robotino UDP transceiver/1(Robotino.ID)
  Rate Transition down-sampling to 50ms/1 -> Robotino UDP transceiver/2(transmit)
  Robotino UDP transceiver/1(receive) -> Unpack1/1
  Status/1 -> Data Type Conversion1/1
  Batteriestand/1 -> Data Type Conversion6/1
  Data Type Conversion6/1 -> Pack/1
  Data Type Conversion1/1 -> Pack/2
  Pack/1 -> Rate Transition down-sampling to 50ms/1

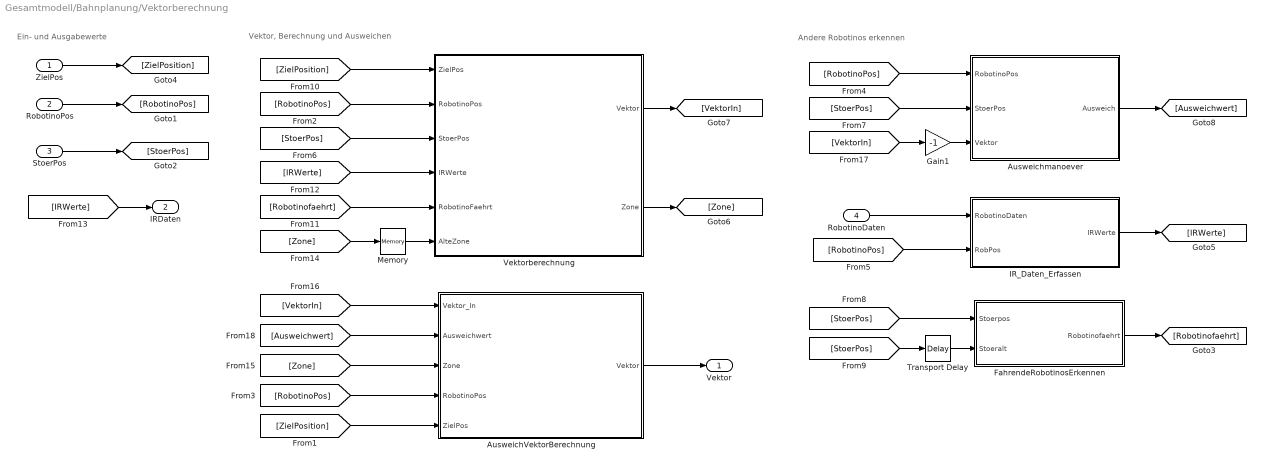
== system Gesamtmodell/Bahnplanung/Vektorberechnung ==
  note: Andere Robotinos erkennen
  note: Ein- und Ausgabewerte
  note: Vektor, Berechnung und Ausweichen
  ZielPos : Inport
  RobotinoPos : Inport  Port=2
  StoerPos : Inport  Port=3
  RobotinoDaten : Inport  Port=4  PortDimensions=15
  AusweichVektorBerechnung : MATLAB Function  TreatAsAtomicUnit=on
  Ausweichmanoever : MATLAB Function  TreatAsAtomicUnit=on
  FahrendeRobotinosErkennen : MATLAB Function  TreatAsAtomicUnit=on
  Gain1 : Gain  Gain=-1
  IR_Daten_Erfassen : MATLAB Function  TreatAsAtomicUnit=on
  Memory : Memory
  Transport Delay : TransportDelay
  Vektorberechnung : MATLAB Function  TreatAsAtomicUnit=on
  Vektor : Outport
  IRDaten : Outport  Port=2
  wires:
  Memory/1 -> Vektorberechnung/6(AlteZone)
  Transport Delay/1 -> FahrendeRobotinosErkennen/2(Stoeralt)
  AusweichVektorBerechnung/1(Vektor) -> Vektor/1
  Gain1/1 -> Ausweichmanoever/3(Vektor)
  RobotinoDaten/1 -> IR_Daten_Erfassen/1(RobotinoDaten)
  [ZielPosition] -> Vektorberechnung/1(ZielPos)
  [ZielPosition] -> AusweichVektorBerechnung/5(ZielPos)
  ZielPos/1 -> [ZielPosition]
  [RobotinoPos] -> AusweichVektorBerechnung/4(RobotinoPos)
  [RobotinoPos] -> Ausweichmanoever/1(RobotinoPos)
  [RobotinoPos] -> IR_Daten_Erfassen/2(RobPos)
  RobotinoPos/1 -> [RobotinoPos]
  [RobotinoPos] -> Vektorberechnung/2(RobotinoPos)
  [StoerPos] -> Vektorberechnung/3(StoerPos)
  [StoerPos] -> Ausweichmanoever/2(StoerPos)
  [StoerPos] -> FahrendeRobotinosErkennen/1(Stoerpos)
  [StoerPos] -> Transport Delay/1
  StoerPos/1 -> [StoerPos]
  [Robotinofaehrt] -> Vektorberechnung/5(RobotinoFaehrt)
  FahrendeRobotinosErkennen/1(Robotinofaehrt) -> [Robotinofaehrt]
  [IRWerte] -> Vektorberechnung/4(IRWerte)
  [IRWerte] -> IRDaten/1
  IR_Daten_Erfassen/1(IRWerte) -> [IRWerte]
  [Zone] -> Memory/1
  [Zone] -> AusweichVektorBerechnung/3(Zone)
  Vektorberechnung/2(Zone) -> [Zone]
  [VektorIn] -> AusweichVektorBerechnung/1(Vektor_In)
  [VektorIn] -> Gain1/1
  Vektorberechnung/1(Vektor) -> [VektorIn]
  [Ausweichwert] -> AusweichVektorBerechnung/2(Ausweichwert)
  Ausweichmanoever/1(Ausweich) -> [Ausweichwert]

== system Gesamtmodell/Regelung1/Receiver ==
  "RoboID " : Inport
  Terminator4 : Terminator
  UDP interface : Subsystem
  autoRobID : MATLAB Function  TreatAsAtomicUnit=on
  x4(psi) : MATLAB Function  TreatAsAtomicUnit=on
  CameraX : Outport
  CameraY : Outport  Port=2
  "CameraPsi " : Outport  Port=3
  CameraSignalValid : Outport  Port=4
  "origAngle " : Outport  Port=5
  UDPDaten : Outport  Port=6
  wires:
  autoRobID/1(pX) -> CameraX/1
  autoRobID/4(enable) -> CameraSignalValid/1
  x4(psi)/1(x4) -> "CameraPsi "/1
  autoRobID/2(pY) -> CameraY/1
  autoRobID/3(psi) -> "origAngle "/1, x4(psi)/1(psi)
  UDP interface/2(UDP data) -> UDPDaten/1, autoRobID/1(udpIn)  "56 elements"
  UDP interface/1(enable) -> Terminator4/1  "1 -> permission granted;        0 -> not granted"
  "RoboID "/1 -> autoRobID/2(robID), UDP interface/1(number of robot)

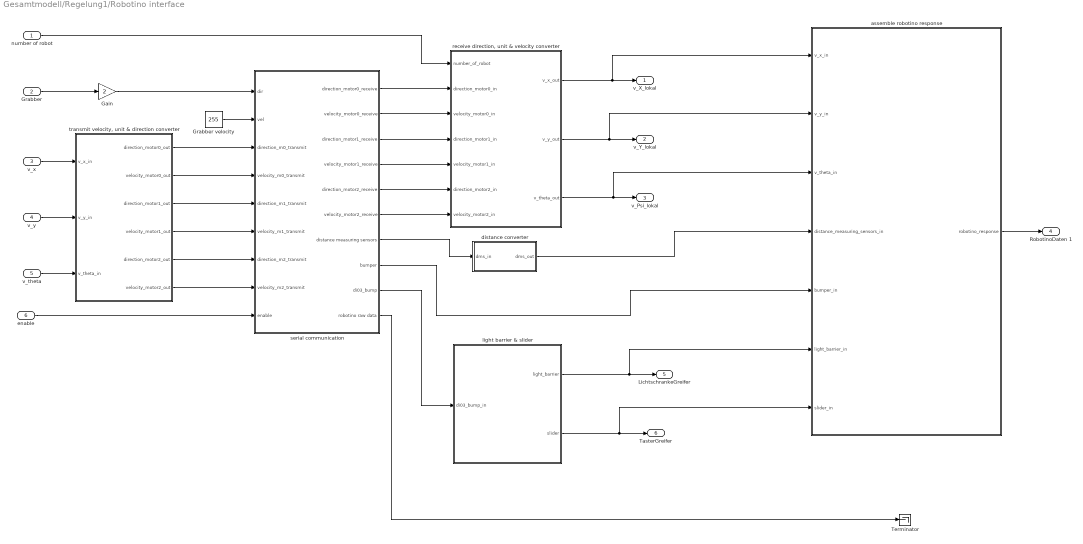
== system Gesamtmodell/Regelung1/Robotino interface ==
  number of robot : Inport
  Grabber : Inport  Port=2
  v_x : Inport  Port=3
  v_y : Inport  Port=4
  v_theta : Inport  Port=5
  enable : Inport  Port=6
  Gain : Gain  Gain=2
  Grabber velocity : Constant  Value=255
  Terminator : Terminator
  assemble robotino response : MATLAB Function  TreatAsAtomicUnit=on
  distance converter : MATLAB Function  TreatAsAtomicUnit=on
  light barrier & slider : MATLAB Function  TreatAsAtomicUnit=on
  "receive direction, unit & velocity converter" : MATLAB Function  TreatAsAtomicUnit=on
  serial communication : Subsystem
  "transmit velocity, unit & direction converter" : MATLAB Function  TreatAsAtomicUnit=on
  v_X_lokal : Outport
  "v_Y_lokal " : Outport  Port=2
  "v_Psi_lokal " : Outport  Port=3
  RobotinoDaten 1 : Outport  Port=4
  LichtschrankeGreifer : Outport  Port=5
  TasterGreifer : Outport  Port=6
  wires:
  "transmit velocity, unit & direction converter"/1(direction_motor0_out) -> serial communication/3(direction_m0_transmit)
  "transmit velocity, unit & direction converter"/2(velocity_motor0_out) -> serial communication/4(velocity_m0_transmit)
  "transmit velocity, unit & direction converter"/3(direction_motor1_out) -> serial communication/5(direction_m1_transmit)
  "transmit velocity, unit & direction converter"/4(velocity_motor1_out) -> serial communication/6(velocity_m1_transmit)
  "transmit velocity, unit & direction converter"/5(direction_motor2_out) -> serial communication/7(direction_m2_transmit)
  "transmit velocity, unit & direction converter"/6(velocity_motor2_out) -> serial communication/8(velocity_m2_transmit)
  v_x/1 -> "transmit velocity, unit & direction converter"/1(v_x_in)
  v_y/1 -> "transmit velocity, unit & direction converter"/2(v_y_in)
  v_theta/1 -> "transmit velocity, unit & direction converter"/3(v_theta_in)
  "receive direction, unit & velocity converter"/2(v_y_out) -> assemble robotino response/2(v_y_in), "v_Y_lokal "/1
  enable/1 -> serial communication/9(enable)
  serial communication/1(direction_motor0_receive) -> "receive direction, unit & velocity converter"/2(direction_motor0_in)
  serial communication/7(distance measuring sensors) -> distance converter/1(dms_in)
  serial communication/10(robotino raw data) -> Terminator/1
  serial communication/9(di03_bump) -> light barrier & slider/1(di03_bump_in)
  "receive direction, unit & velocity converter"/1(v_x_out) -> assemble robotino response/1(v_x_in), v_X_lokal/1
  "receive direction, unit & velocity converter"/3(v_theta_out) -> assemble robotino response/3(v_theta_in), "v_Psi_lokal "/1
  Grabber/1 -> Gain/1
  Gain/1 -> serial communication/1(dir)
  distance converter/1(dms_out) -> assemble robotino response/4(distance_measuring_sensors_in)
  light barrier & slider/2(slider) -> TasterGreifer/1, assemble robotino response/7(slider_in)
  light barrier & slider/1(light_barrier) -> assemble robotino response/6(light_barrier_in), LichtschrankeGreifer/1
  serial communication/8(bumper) -> assemble robotino response/5(bumper_in)
  serial communication/2(velocity_motor0_receive) -> "receive direction, unit & velocity converter"/3(velocity_motor0_in)
  serial communication/3(direction_motor1_receive) -> "receive direction, unit & velocity converter"/4(direction_motor1_in)
  serial communication/4(velocity_motor1_receive) -> "receive direction, unit & velocity converter"/5(velocity_motor1_in)
  serial communication/5(direction_motor2_receive) -> "receive direction, unit & velocity converter"/6(direction_motor2_in)
  serial communication/6(velocity_motor2_receive) -> "receive direction, unit & velocity converter"/7(velocity_motor2_in)
  Grabber velocity/1 -> serial communication/2(vel)
  number of robot/1 -> "receive direction, unit & velocity converter"/1(number_of_robot)
  assemble robotino response/1(robotino_response) -> RobotinoDaten 1/1

== system Gesamtmodell/Regelung1/Signal Builder ==
  Demux : Demux  Tag=STV Demux  Outputs=3
  FromWs : FromWorkspace  Tag=STV FromWs  VariableName=tuvar  SampleTime=0
      SigBuilderData=|
      | common.afterFinalStr = 'Extrapolate'
      | common.sampleTime = 0
      | dataSet.timeRange = [0 25]
      | dataSet.name = 'Group 1'
      | sbobj.Groups.Name = 'Group 1'
      | sbobj.Groups.Signals(1).Name = 'X Pos'
      | sbobj.Groups.Signals(1).XData = [0 5 7.5 10 12.5 25]
      | sbobj.Groups.Signals(1).YData = [5500 5500 6500 6500 5500 5500]
      | sbobj.Groups.Signals(2).Name = 'Y Pos'
      | sbobj.Groups.Signals(2).XData = [0 2.5 5 7.5 10 25]
      | sbobj.Groups.Signals(2).YData = [1000 1000 2000 2000 1000 1000]
      | sbobj.Groups.Signals(3).Name = 'Psi'
      | sbobj.Groups.Signals(3).XData = [0 2.5 5 7.5 10 20 25]
      | sbobj.Groups.Signals(3).YData = [0 0 3.14159265359 3.14159265359 0 0 0]
      | sbobj.Groups.TimeRange = [0 25]
  X Pos : Outport  Tag=STV Outport
  Y Pos : Outport  Tag=STV Outport  Port=2
  Psi : Outport  Tag=STV Outport  Port=3
  wires:
  FromWs/1 -> Demux/1
  Demux/1 -> X Pos/1
  Demux/2 -> Y Pos/1
  Demux/3 -> Psi/1

== system Gesamtmodell/Regelung1/Signal Builder1 ==
  Demux : Demux  Tag=STV Demux  Outputs=3
  FromWs : FromWorkspace  Tag=STV FromWs  VariableName=tuvar  SampleTime=0
  X Pos : Outport  Tag=STV Outport
  Y Pos : Outport  Tag=STV Outport  Port=2
  Psi : Outport  Tag=STV Outport  Port=3
  wires:
  FromWs/1 -> Demux/1
  Demux/1 -> X Pos/1
  Demux/2 -> Y Pos/1
  Demux/3 -> Psi/1

== system Gesamtmodell/Regelung1/Signal Builder2 ==
  Demux : Demux  Tag=STV Demux  Outputs=3
  FromWs : FromWorkspace  Tag=STV FromWs  VariableName=tuvar  SampleTime=0
      SigBuilderData=|
      | common.afterFinalStr = 'Extrapolate'
      | common.sampleTime = 0
      | dataSet.timeRange = [0 25]
      | dataSet.name = 'Group 1'
      | sbobj.Groups.Name = 'Group 1'
      | sbobj.Groups.Signals(1).Name = 'X Pos'
      | sbobj.Groups.Signals(1).XData = [0 2.5 5 10 12.5 25]
      | sbobj.Groups.Signals(1).YData = [5500 5500 5500 5500 5500 5500]
      | sbobj.Groups.Signals(2).Name = 'Y Pos'
      | sbobj.Groups.Signals(2).XData = [0 2.5 5 10 12.5 15 25]
      | sbobj.Groups.Signals(2).YData = [1000 1000 2000 2000 1000 1000 1000]
      | sbobj.Groups.Signals(3).Name = 'Psi'
      | sbobj.Groups.Signals(3).XData = [0 6 10 20 23.72 25]
      | sbobj.Groups.Signals(3).YData = [0 0 0 0 0 0]
      | sbobj.Groups.TimeRange = [0 25]
  X Pos : Outport  Tag=STV Outport
  Y Pos : Outport  Tag=STV Outport  Port=2
  Psi : Outport  Tag=STV Outport  Port=3
  wires:
  FromWs/1 -> Demux/1
  Demux/1 -> X Pos/1
  Demux/2 -> Y Pos/1
  Demux/3 -> Psi/1

== system Gesamtmodell/Regelung1/Signal Builder3 ==
  Demux : Demux  Tag=STV Demux  Outputs=3
  FromWs : FromWorkspace  Tag=STV FromWs  VariableName=tuvar  SampleTime=0
      SigBuilderData=|
      | common.afterFinalStr = 'Extrapolate'
      | common.sampleTime = 0
      | dataSet.timeRange = [0 45]
      | dataSet.name = 'Group 1'
      | sbobj.Groups.Name = 'Group 1'
      | sbobj.Groups.Signals(1).Name = 'X Pos'
      | sbobj.Groups.Signals(1).XData = [0 5 10 15 20 24.95 30.05 35 40 45]
      | sbobj.Groups.Signals(1).YData = [1400 1400 1900 2400 2400 2400 2400 1900 1400 1400]
      | sbobj.Groups.Signals(2).Name = 'Y Pos'
      | sbobj.Groups.Signals(2).XData = [0 0.55 5 10 15 19.95 25 29.95 35 40 45]
      | sbobj.Groups.Signals(2).YData = [1000 1000 1500 1500 1500 1500 1250 1000 1000 1000 1000]
      | sbobj.Groups.Signals(3).Name = 'Psi'
      | sbobj.Groups.Signals(3).XData = [0 5 10 15 20 25 30 35.1 40 45]
      | sbobj.Groups.Signals(3).YData = [1.5708 1.5708 6.28318530718 3.14 0 0 -3.14159265359 3.14159265359 0 0]
      | sbobj.Groups.TimeRange = [0 45]
  X Pos : Outport  Tag=STV Outport
  Y Pos : Outport  Tag=STV Outport  Port=2
  Psi : Outport  Tag=STV Outport  Port=3
  wires:
  Demux/3 -> Psi/1
  Demux/2 -> Y Pos/1
  Demux/1 -> X Pos/1
  FromWs/1 -> Demux/1

== system Gesamtmodell/Regelung1/Signal Builder4 ==
  Demux : Demux  Tag=STV Demux  Outputs=3
  FromWs : FromWorkspace  Tag=STV FromWs  VariableName=tuvar  SampleTime=0
      SigBuilderData=|
      | common.afterFinalStr = 'Extrapolate'
      | common.sampleTime = 0
      | dataSet.timeRange = [0 45]
      | dataSet.name = 'Group 1'
      | sbobj.Groups.Name = 'Group 1'
      | sbobj.Groups.Signals(1).Name = 'X Pos'
      | sbobj.Groups.Signals(1).XData = [0 5 10 15 20 24.95 30.05 35 40 45]
      | sbobj.Groups.Signals(1).YData = [3400 3400 3900 4400 4400 4400 4400 3900 3400 3400]
      | sbobj.Groups.Signals(2).Name = 'Y Pos'
      | sbobj.Groups.Signals(2).XData = [0 0.55 5 10 15 19.95 25 29.95 35 40 45]
      | sbobj.Groups.Signals(2).YData = [1000 1000 1500 1500 1500 1500 1250 1000 1000 1000 1000]
      | sbobj.Groups.Signals(3).Name = 'Psi'
      | sbobj.Groups.Signals(3).XData = [0 5 10 15 20 25 30 35.1 40 45]
      | sbobj.Groups.Signals(3).YData = [1.5708 1.5708 6.28318530718 3.14 0 0 -3.14159265359 3.14159265359 0 0]
      | sbobj.Groups.TimeRange = [0 45]
  X Pos : Outport  Tag=STV Outport
  Y Pos : Outport  Tag=STV Outport  Port=2
  Psi : Outport  Tag=STV Outport  Port=3
  wires:
  Demux/3 -> Psi/1
  Demux/2 -> Y Pos/1
  Demux/1 -> X Pos/1
  FromWs/1 -> Demux/1

== system Gesamtmodell/Regelung1/Signal Builder5 ==
  Demux : Demux  Tag=STV Demux  Outputs=3
  FromWs : FromWorkspace  Tag=STV FromWs  VariableName=tuvar  SampleTime=0
      SigBuilderData=|
      | common.afterFinalStr = 'Extrapolate'
      | common.sampleTime = 0
      | dataSet.timeRange = [0 45]
      | dataSet.name = 'Group 1'
      | sbobj.Groups.Name = 'Group 1'
      | sbobj.Groups.Signals(1).Name = 'X Pos'
      | sbobj.Groups.Signals(1).XData = [0 5 10 15 20 24.95 30.05 35 40 45]
      | sbobj.Groups.Signals(1).YData = [5300 4850 4100 3200 2850 2250 1900 1650 1400 750]
      | sbobj.Groups.Signals(2).Name = 'Y Pos'
      | sbobj.Groups.Signals(2).XData = [0 0.55 5 10 15 19.95 25 29.95 35 40 45]
      | sbobj.Groups.Signals(2).YData = [3450 3450 3450 3450 3450 3450 3450 3450 3450 3450 3450]
      | sbobj.Groups.Signals(3).Name = 'Psi'
      | sbobj.Groups.Signals(3).XData = [0 5 10 15 20 25 30 35.1 40 45]
      | sbobj.Groups.Signals(3).YData = [1.57079632679 1.56 1.54 0 0 -1.57079632679 -1.5 -1.46 0 0]
      | sbobj.Groups.TimeRange = [0 45]
  X Pos : Outport  Tag=STV Outport
  Y Pos : Outport  Tag=STV Outport  Port=2
  Psi : Outport  Tag=STV Outport  Port=3
  wires:
  Demux/3 -> Psi/1
  Demux/2 -> Y Pos/1
  Demux/1 -> X Pos/1
  FromWs/1 -> Demux/1

== system Gesamtmodell/Regelung1/Stellgrößen- beschränkung  ==
  note: in rad/sec
  note: in mm/sec
  note: in mm/sec
  vX : Inport
  vY : Inport  Port=2
  vPsi : Inport  Port=3
  "Beschraenkung " : MATLAB Function  TreatAsAtomicUnit=on
  MaxStellR : Constant  Value=5
  MaxStellT : Constant  Value=400
  vXlim : Outport
  vYlim : Outport  Port=2
  vPsiLim : Outport  Port=3
  wires:
  MaxStellT/1 -> "Beschraenkung "/1(MaxStellT)
  "Beschraenkung "/1(X) -> vXlim/1
  "Beschraenkung "/2(Y) -> vYlim/1
  "Beschraenkung "/3(Theta) -> vPsiLim/1
  MaxStellR/1 -> "Beschraenkung "/2(MaxStellR)
  vX/1 -> "Beschraenkung "/3(x)
  vY/1 -> "Beschraenkung "/4(y)
  vPsi/1 -> "Beschraenkung "/5(theta)

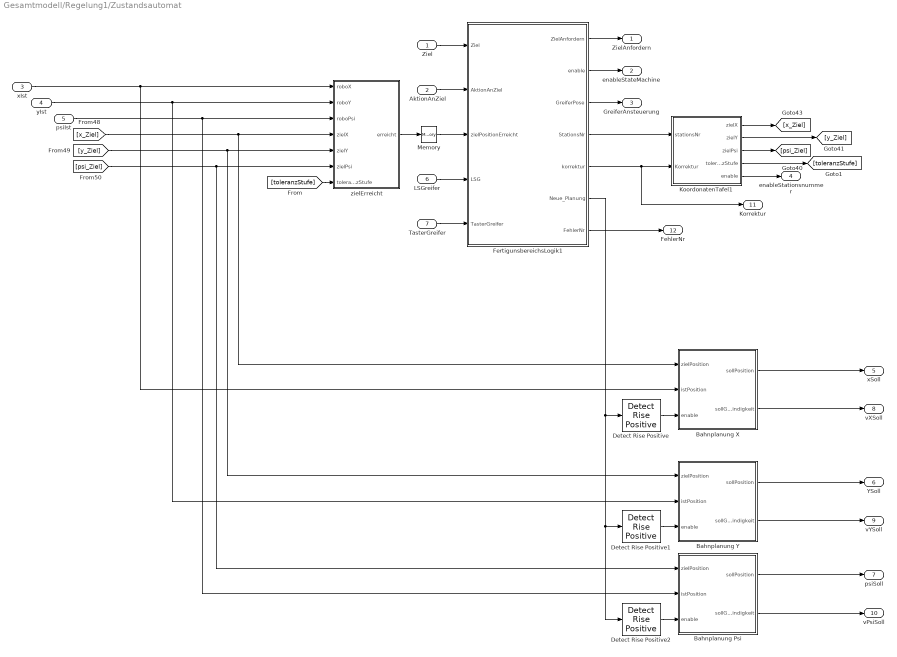
== system Gesamtmodell/Regelung1/Zustandsautomat ==
  "Ziel " : Inport
  AktionAnZiel : Inport  Port=2
  xIst : Inport  Port=3
  yIst : Inport  Port=4
  psiIst : Inport  Port=5
  "LSGreifer " : Inport  Port=6
  "TasterGreifer " : Inport  Port=7
  Bahnplanung Psi : MATLAB Function  TreatAsAtomicUnit=on
  Bahnplanung X : MATLAB Function  TreatAsAtomicUnit=on
  Bahnplanung Y : MATLAB Function  TreatAsAtomicUnit=on
  Detect Rise Positive : simulink/Logic and Bit Operations/Detect Rise Positive  vinit=0  InputProcessing=Inherited  OutDataTypeStr=boolean
  Detect Rise Positive1 : simulink/Logic and Bit Operations/Detect Rise Positive  vinit=0  InputProcessing=Inherited  OutDataTypeStr=boolean
  Detect Rise Positive2 : simulink/Logic and Bit Operations/Detect Rise Positive  vinit=0  InputProcessing=Inherited  OutDataTypeStr=boolean
  FertigunsbereichsLogik1 : Stateflow chart  TreatAsAtomicUnit=on
  KoordonatenTafel1 : MATLAB Function  TreatAsAtomicUnit=on
  Memory : Memory
  zielErreicht : MATLAB Function  TreatAsAtomicUnit=on
  ZielAnfordern : Outport
  enableStateMachine : Outport  Port=2
  GreiferAnsteuerung : Outport  Port=3
  enableStationsnummer : Outport  Port=4
  xSoll : Outport  Port=5
  YSoll : Outport  Port=6
  psiSoll : Outport  Port=7
  vXSoll : Outport  Port=8
  vYSoll : Outport  Port=9
  vPsiSoll : Outport  Port=10
  Korrektur : Outport  Port=11
  FehlerNr : Outport  Port=12
  wires:
  FertigunsbereichsLogik1/7(FehlerNr) -> FehlerNr/1
  "TasterGreifer "/1 -> FertigunsbereichsLogik1/5(TasterGreifer)
  Bahnplanung Psi/2(sollGeschwindigkeit) -> vPsiSoll/1
  Bahnplanung Psi/1(sollPosition) -> psiSoll/1
  Bahnplanung Y/2(sollGeschwindigkeit) -> vYSoll/1
  Bahnplanung Y/1(sollPosition) -> YSoll/1
  Bahnplanung X/1(sollPosition) -> xSoll/1
  Detect Rise Positive/1 -> Bahnplanung X/3(enable)
  [y_Ziel] -> zielErreicht/5(zielY), Bahnplanung Y/1(zielPosition)
  Detect Rise Positive1/1 -> Bahnplanung Y/3(enable)
  Detect Rise Positive2/1 -> Bahnplanung Psi/3(enable)
  FertigunsbereichsLogik1/6(Neue_Planung) -> Detect Rise Positive1/1, Detect Rise Positive2/1, Detect Rise Positive/1
  xIst/1 -> zielErreicht/1(roboX), Bahnplanung X/2(istPosition)
  [x_Ziel] -> zielErreicht/4(zielX), Bahnplanung X/1(zielPosition)
  yIst/1 -> zielErreicht/2(roboY), Bahnplanung Y/2(istPosition)
  [psi_Ziel] -> zielErreicht/6(zielPsi), Bahnplanung Psi/1(zielPosition)
  psiIst/1 -> zielErreicht/3(roboPsi), Bahnplanung Psi/2(istPosition)
  KoordonatenTafel1/3(zielPsi) -> [psi_Ziel]
  KoordonatenTafel1/2(zielY) -> [y_Ziel]
  KoordonatenTafel1/1(zielX) -> [x_Ziel]
  FertigunsbereichsLogik1/3(GreiferPose) -> GreiferAnsteuerung/1
  FertigunsbereichsLogik1/1(ZielAnfordern) -> ZielAnfordern/1
  zielErreicht/1(erreicht) -> Memory/1
  "Ziel "/1 -> FertigunsbereichsLogik1/1(Ziel)
  Memory/1 -> FertigunsbereichsLogik1/3(zielPositionErreicht)
  FertigunsbereichsLogik1/4(StationsNr) -> KoordonatenTafel1/1(stationsNr)
  FertigunsbereichsLogik1/2(enable) -> enableStateMachine/1
  AktionAnZiel/1 -> FertigunsbereichsLogik1/2(AktionAnZiel)
  KoordonatenTafel1/5(enable) -> enableStationsnummer/1
  "LSGreifer "/1 -> FertigunsbereichsLogik1/4(LSG)
  KoordonatenTafel1/4(toleranzStufe) -> [toleranzStufe]
  [toleranzStufe] -> zielErreicht/7(toleranzStufe)
  Bahnplanung X/2(sollGeschwindigkeit) -> vXSoll/1
  FertigunsbereichsLogik1/5(korrektur) -> Korrektur/1, KoordonatenTafel1/2(Korrektur)

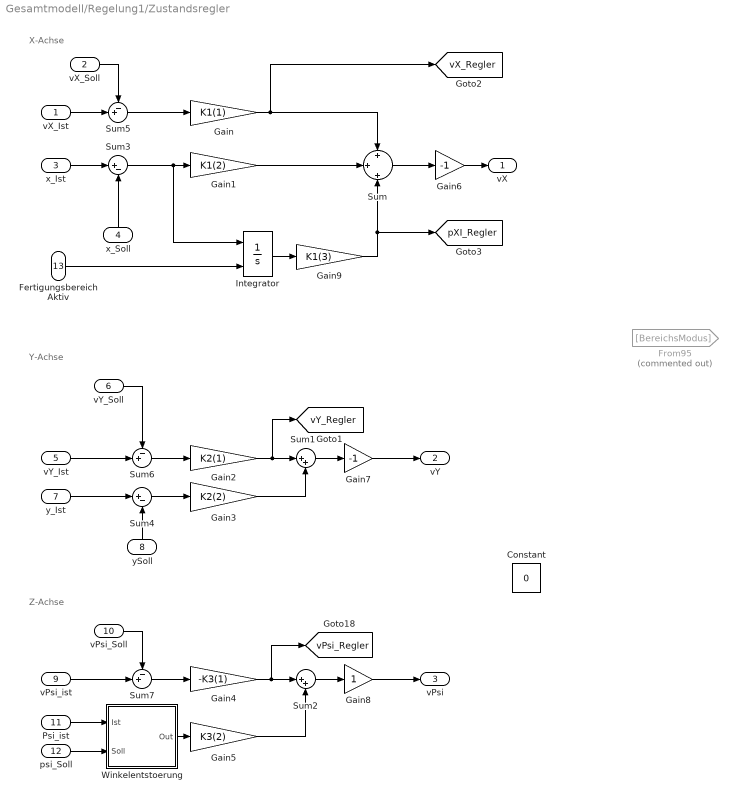
== system Gesamtmodell/Regelung1/Zustandsregler ==
  note: Z-Achse
  note: Y-Achse
  note: X-Achse
  vX_Ist : Inport
  "vX_Soll " : Inport  Port=2
  x_Ist : Inport  Port=3
  x_Soll : Inport  Port=4
  vY_Ist : Inport  Port=5
  "vY_Soll " : Inport  Port=6
  y_Ist : Inport  Port=7
  ySoll : Inport  Port=8
  vPsi_ist : Inport  Port=9
  vPsi_Soll : Inport  Port=10
  Psi_ist : Inport  Port=11
  "psi_Soll " : Inport  Port=12
  Fertigungsbereich Aktiv : Inport  Port=13
  Constant : Constant  Value=0
  From95 : From  Commented=on  GotoTag=BereichsModus
  Gain : Gain  Gain=K1(1)
  Gain1 : Gain  Gain=K1(2)
  Gain2 : Gain  Gain=K2(1)
  Gain3 : Gain  Gain=K2(2)
  Gain4 : Gain  Gain=-K3(1)
  Gain5 : Gain  Gain=K3(2)
  Gain6 : Gain  Gain=-1
  Gain7 : Gain  Gain=-1
  Gain8 : Gain
  Gain9 : Gain  Gain=K1(3)
  Integrator : Integrator  ExternalReset=rising
  Sum : Sum  Inputs=+|+|+
  Sum1 : Sum  Inputs=|++
  Sum2 : Sum  Inputs=|++
  Sum3 : Sum  Inputs=|+-
  Sum4 : Sum  Inputs=|+-
  Sum5 : Sum  Inputs=-+|
  Sum6 : Sum  Inputs=-+|
  Sum7 : Sum  Inputs=-+|
  Winkelentstoerung : MATLAB Function  TreatAsAtomicUnit=on
  vX : Outport
  vY : Outport  Port=2
  "vPsi " : Outport  Port=3
  tag scope: pXI_Regler=global, vPsi_Regler=global, vX_Regler=global, vY_Regler=global
  wires:
  Fertigungsbereich Aktiv/1 -> Integrator/2
  Gain/1 -> [vX_Regler], Sum/1
  Gain1/1 -> Sum/2
  Gain2/1 -> [vY_Regler], Sum1/1
  Gain3/1 -> Sum1/2
  Gain4/1 -> Sum2/1, [vPsi_Regler]
  Gain5/1 -> Sum2/2
  Sum1/1 -> Gain7/1
  Sum/1 -> Gain6/1
  x_Ist/1 -> Sum3/1
  Sum3/1 -> Integrator/1, Gain1/1
  y_Ist/1 -> Sum4/1
  Sum4/1 -> Gain3/1
  Gain6/1 -> vX/1
  Gain7/1 -> vY/1
  vPsi_ist/1 -> Sum7/2
  Sum2/1 -> Gain8/1
  Gain8/1 -> "vPsi "/1
  Psi_ist/1 -> Winkelentstoerung/1(Ist)
  vX_Ist/1 -> Sum5/2
  Sum5/1 -> Gain/1
  vY_Ist/1 -> Sum6/2
  Sum6/1 -> Gain2/1
  "vX_Soll "/1 -> Sum5/1
  "vY_Soll "/1 -> Sum6/1
  Sum7/1 -> Gain4/1
  vPsi_Soll/1 -> Sum7/1
  x_Soll/1 -> Sum3/2
  ySoll/1 -> Sum4/2
  "psi_Soll "/1 -> Winkelentstoerung/2(Soll)
  Winkelentstoerung/1(Out) -> Gain5/1
  Integrator/1 -> Gain9/1
  Gain9/1 -> [pXI_Regler], Sum/3

== system Gesamtmodell/Regelung1/getRobotinoID ==
  note: Executing only once at start after 10ms
  Step : Step  Time=0.01  SampleTime=0
  getIDfromFlash : Subsystem
  Robotino.ID : Outport
  wires:
  Step/1 -> getIDfromFlash/Trigger
  getIDfromFlash/1(RobotinoID) -> Robotino.ID/1
